simulink model "base_python_example_23a"  (R2023b)
settings: Solver=FixedStepAuto  StartTime=0.0  StopTime=20  FixedStep=0.2  RelTol=1e-3
InitFcn:
  | coeffStds = [0.002995595096857,0.076600147330248,0.631288082601997,0.002600128777275,0.073641936476251,0.984567040148445];
  | coeffMeans = [-1.939450143265110e-04,1.557727430093527e-04,1.473991581706893,-1.909623131136531e-04,0.004474616468621,-1.378729416735388];
  | Isize = single(zeros(227,227));
libraries: HumanDetection x1
settings Model: PauseTimes=0.1  Creator=lnarasim  LastModifiedBy=ydebray
settings SolverCC: AlgebraicLoopSolver=TrustRegion
settings DataIOCC: ReturnWorkspaceOutputs=off
settings DebuggingCC: UnconnectedInputMsg=warning  UnconnectedOutputMsg=warning  UnconnectedLineMsg=warning  ArithmeticOperatorsInVariantConditions=warning
settings ModelReferenceCC: EnableRefExpFcnMdlSchedulingChecks=on
settings SFSimCC: SimUseLocalCustomCode=off  DefaultCustomCodeFunctionArrayLayout=Row-major  CustomCodeUndefinedFunction=UseInterfaceOnly
settings RTWCC: RTWUseLocalCustomCode=off  DLArmComputeVersion=19.05

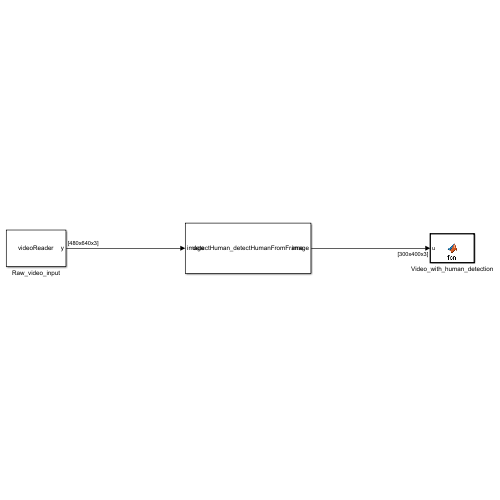
[thumbnail: Simulink's stored preview of the top-level diagram]
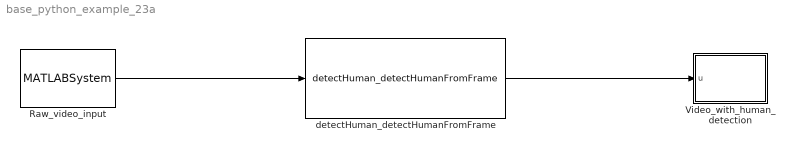
== system base_python_example_23a ==
  Raw_video_input : MATLABSystem  System=videoReader  SimulateUsing=Interpreted execution
      mask Type: videoReader
      mask Display:
      | disp('videoReader');
      | port_label('output',1,'y');
  Video_with_human_detection : MATLAB Function  TreatAsAtomicUnit=on
  detectHuman_detectHumanFromFrame : HumanDetection/detectHuman_detectHumanFromFrame
  wires:
  Raw_video_input/1 -> detectHuman_detectHumanFromFrame/1
  detectHuman_detectHumanFromFrame/1 -> Video_with_human_detection/1(u)

== matlab function base_python_example_23a/Video_with_human_detection ==
  data: u input
function fcn(u)
    coder.extrinsic('imagesc');
    imagesc(u);
    drawnow
